simulink model "PlantEsempio1"  (Simulink 6.2)
settings: Solver=ode3  StartTime=0.0  StopTime=inf  RelTol=1e-3
settings Model: LastModifiedBy=Administrator
settings DebuggingCC: SolverPrmCheckMsg=warning

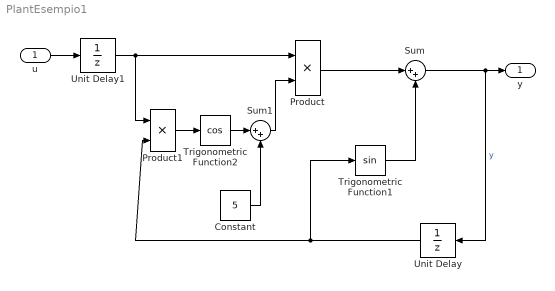
== system PlantEsempio1 ==
  u : Inport  Port=1  LatchInput=off
  Constant : Constant  Value=5
  Product : Product  RndMeth=Zero
  Product1 : Product  RndMeth=Zero
  Sum : Sum  Inputs=|++
  Sum1 : Sum  Inputs=|++
  Trigonometric Function1 : Trigonometry
  Trigonometric Function2 : Trigonometry  Operator=cos
  Unit Delay : UnitDelay  Orientation=left
  Unit Delay1 : UnitDelay
  y : Outport
  wires:
  Unit Delay/1 -> Trigonometric Function1/1, Product1/2
  Product/1 -> Sum/1
  Trigonometric Function1/1 -> Sum/2
  Sum/1 -> Unit Delay/1, y/1  "y"
  u/1 -> Unit Delay1/1
  Product1/1 -> Trigonometric Function2/1
  Trigonometric Function2/1 -> Sum1/1
  Sum1/1 -> Product/2
  Constant/1 -> Sum1/2
  Unit Delay1/1 -> Product1/1, Product/1
